simulink model "Feedback_Control"  (R2023b)
settings: Solver=ode45  StartTime=0.0  StopTime=runtime  RelTol=1e-3
values from neighbouring files (symbols this model uses):
  den = sym2poly(den)    [miniproject1.m]
  dist = 0    [miniproject1.m]
  k = 1000    [miniproject1.m]
  noise = 0    [miniproject1.m]
  num = sym2poly(num)    [miniproject1.m]
  ref = 0    [miniproject1.m]
  sinwave = 0    [miniproject1.m]
undefined symbols (not defined in the file or in its folder): den_controller, num_controller
settings Model: Creator=e7nel  LastModifiedBy=e7nel
settings DataIOCC: SaveOutput=off  SignalLogging=off  DSMLogging=off  SaveTime=off  ReturnWorkspaceOutputs=off
settings ModelReferenceCC: EnableRefExpFcnMdlSchedulingChecks=on

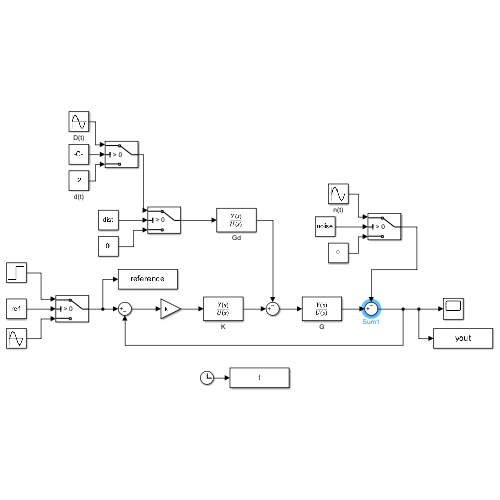
[thumbnail: Simulink's stored preview of the top-level diagram]
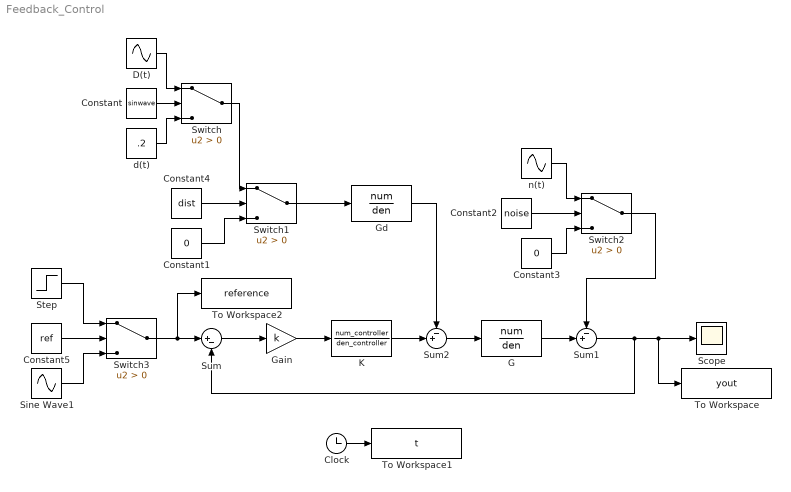
== system Feedback_Control ==
  Clock : Clock
  Constant : Constant  Value=sinwave
  Constant1 : Constant  Value=0
  Constant2 : Constant  Value=noise
  Constant3 : Constant  Value=0
  Constant4 : Constant  Value=dist
  Constant5 : Constant  Value=ref
  D(t) : Sin  Amplitude=.2  Frequency=2  SampleTime=0
  G : TransferFcn  Numerator=num  Denominator=den  ParameterTunability=Optimized
  Gain : Gain  Gain=k
  Gd : TransferFcn  Numerator=num  Denominator=den
  K : TransferFcn  Numerator=num_controller  Denominator=den_controller
  Scope : Scope
  Sine Wave1 : Sin  Amplitude=3  Frequency=5  SampleTime=0
  Step : Step  Time=.01  SampleTime=0
  Sum : Sum  Inputs=|+-
  Sum1 : Sum  Inputs=-+|
  Sum2 : Sum  Inputs=-+|
  Switch{,1..3} (4 alike) : Switch  Criteria=u2 > Threshold  SaturateOnIntegerOverflow=off  InputSameDT=off
  To Workspace : ToWorkspace  VariableName=yout  SampleTime=-1
      settings: Save2DSignal=2-D array (concatenate along first dimension)
  To Workspace1 : ToWorkspace  VariableName=t  SampleTime=-1
      settings: Save2DSignal=2-D array (concatenate along first dimension)
  To Workspace2 : ToWorkspace  VariableName=reference  SampleTime=-1
      settings: Save2DSignal=2-D array (concatenate along first dimension)
  d(t) : Constant  Value=.2
  n(t) : Sin  Frequency=20  SampleTime=0
  wires:
  n(t)/1 -> Switch2/1
  Clock/1 -> To Workspace1/1
  Sum2/1 -> G/1
  Constant/1 -> Switch/2
  Constant2/1 -> Switch2/2
  Constant3/1 -> Switch2/3
  G/1 -> Sum1/2
  Switch2/1 -> Sum1/1
  Sum1/1 -> Sum/2, To Workspace/1, Scope/1
  d(t)/1 -> Switch/3
  D(t)/1 -> Switch/1
  Switch3/1 -> To Workspace2/1, Sum/1
  Sine Wave1/1 -> Switch3/3
  Step/1 -> Switch3/1
  Constant5/1 -> Switch3/2
  Sum/1 -> Gain/1
  Constant1/1 -> Switch1/3
  Constant4/1 -> Switch1/2
  Switch/1 -> Switch1/1
  Switch1/1 -> Gd/1
  K/1 -> Sum2/2
  Gain/1 -> K/1
  Gd/1 -> Sum2/1
